simulink model "chap5_10sim"  (Simulink 7.7)
settings: Solver=ode45  StartTime=0.0  StopTime=20  FixedStep=0.001  RelTol=1e-3
libraries: simulink x1
settings Model: Creator=hp  LastModifiedBy=ljk  ExtModeTrigMode=oneshot  ExtModeArmWhenConnect=off
settings DataIOCC: LimitDataPoints=off  SignalLoggingName=sigsOut
settings OptimizationCC: BooleanDataType=off  InitFltsAndDblsToZero=on
settings DebuggingCC: SaveWithParameterizedLinksMsg=none  SignalResolutionControl=TryResolveAllWithWarning  SolverPrmCheckMsg=none  MultiTaskDSMMsg=warning  MultiTaskCondExecSysMsg=none  StrictBusMsg=None
settings HardwareCC: TargetUnknown=on
settings RTWCC: IncludeERTFirstTime=on
settings GRTTargetCC: TargetFcnLib=ansi_tfl_tmw.mat

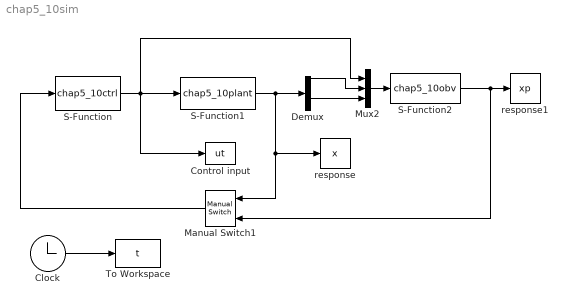
== system chap5_10sim ==
  Clock : Clock
      settings: Decimation=10
  Control input : ToWorkspace  VariableName=ut  SampleTime=-1  SaveFormat=Array
  Demux : Demux
  Manual Switch1 : simulink/Signal Routing/Manual Switch  SystemSampleTime=-1  sw=0  action=0  varsize=off
  Mux2 : Mux  Inputs=3
  S-Function : S-Function  FunctionName=chap5_10ctrl  EnableBusSupport=off
  S-Function1 : S-Function  FunctionName=chap5_10plant  EnableBusSupport=off
  S-Function2 : S-Function  FunctionName=chap5_10obv  EnableBusSupport=off
  To Workspace : ToWorkspace  VariableName=t  SampleTime=-1  SaveFormat=Array
  response : ToWorkspace  VariableName=x  SampleTime=-1  SaveFormat=Array
  response1 : ToWorkspace  VariableName=xp  SampleTime=-1  SaveFormat=Array
  wires:
  S-Function/1 -> S-Function1/1, Mux2/1, Control input/1
  Clock/1 -> To Workspace/1
  S-Function2/1 -> Manual Switch1/2, response1/1
  Mux2/1 -> S-Function2/1
  S-Function1/1 -> Demux/1, response/1, Manual Switch1/1
  Demux/1 -> Mux2/2
  Demux/3 -> Mux2/3
  Manual Switch1/1 -> S-Function/1
